simulink subsystem "Simulation"  (R2025b)
settings: Solver=VariableStepAuto  StartTime=0.0  StopTime=10.0  RelTol=1e-3
undefined symbols (not defined in the file or in its folder): angular_velocity, AUV, data, data_SL_Info, elevation, fractalcoef, heading, height, linear_acceleration, orientation, Sim3dSensor, Simple, T200, thruster_pose, width, x_vel_btm, XYZ, y_vel_btm, z_vel_btm
libraries: ros2lib x15, sim3dlib x7, robotcorelib x5, AUVLib x4, aerolib6dof2 x2, sim3dcameralib x2, matrix_library x1, mspsensorlib x1, aerolibutil x1, mspfiltlib x1
(part 1 of 2)
settings Model: Creator=ubuntu  LastModifiedBy=ubuntu

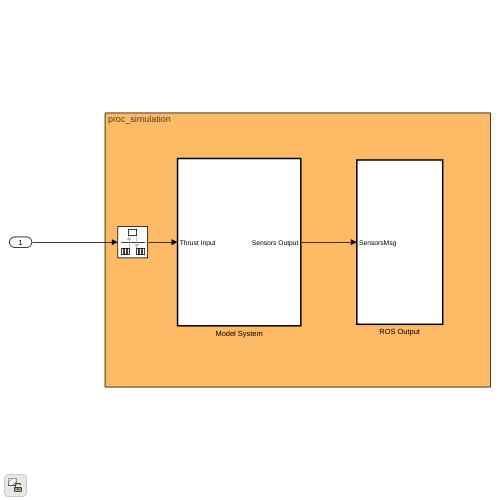
[thumbnail: Simulink's stored preview of the top-level diagram]
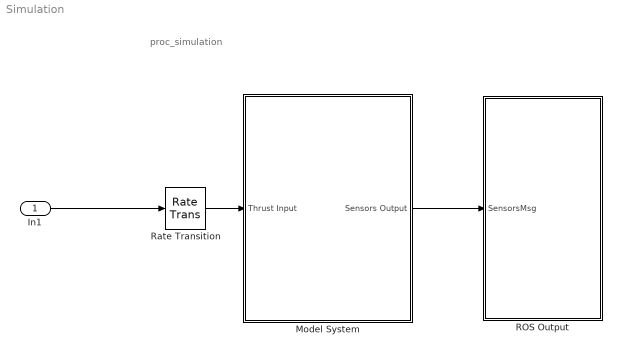
== system Simulation ==
  note: proc_simulation
  In1 : Inport
  Model System : Subsystem  TreatAsAtomicUnit=on
  ROS Output : Subsystem  TreatAsAtomicUnit=on
  Rate Transition : RateTransition  OutPortSampleTime=0.05
  wires:
  Model System/1(Sensors Output) -> ROS Output/1(SensorsMsg)
  In1/1 -> Rate Transition/1
  Rate Transition/1 -> Model System/1(Thrust Input)

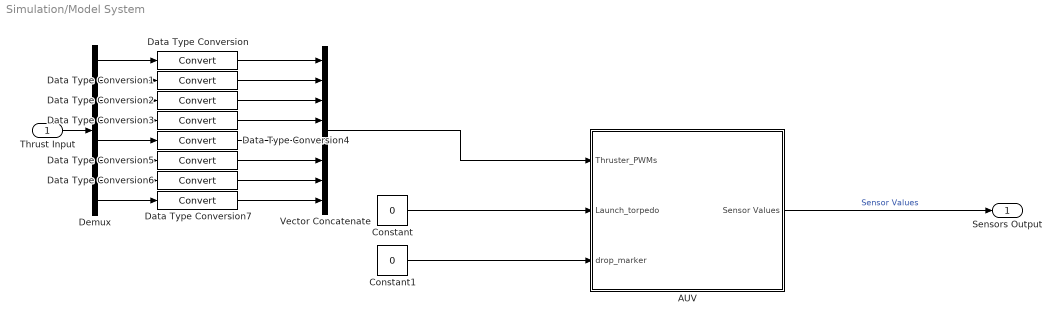
== system Simulation/Model System ==
  Thrust Input : Inport
  AUV : Subsystem  mask(RoboSub){SourceFile=./src/virtual-robosub/fbx files/AUV2.stl, AUV_cob=[0.01, -0.02, -0.10], AUV_height=AUV.Body.hulldiameter, AUV_vol=0.0365, AUV_inertia=AUV.Body.Inertia, AUV_mass=31.42, AUV_pos=[-142 -142 -1], AUV_orientation=[0 0 pi/2], thruster_pose=thruster_pose, AUV_Voltage=16V, nThrusters=8, Hy=Simple, lin_coeff=diag([ 150,200,153]), quad_coeff=diag([ 11.7, 8.2, 7.56]), ang_coeff=diag([ 33, 23, 50]), CMK=AUV.Coeff.CMM, CMM=AUV.Coeff.CMN, CMN=AUV.Coeff.CMK, CZ=AUV.Coeff.CZ, CY=AUV.Coeff.CY, CX=AUV.Coeff.CX, betaR=AUV.IncRange.beta_vec, alphaR=AUV.IncRange.alpha_vec, ang_coeff_c=diag([10, 80, 80]), d_cam_pos=[0 0 -0.26], d_orientation=[0 90 0], SemanticOutportEnabled=off, DepthOutportEnabled=off, TangentialDistortion=[0, 0], RadialDistortion=[0, 0], ImageSize=[720, 1280], OpticalCenter=[640, 360], FocalLength=[1109, 1109], f_cam_pos=[0.5, 0, 0], f_orientation=[0 0 0], SemanticOutportEnabled_f=off, DepthOutportEnabled_f=on, TangentialDistortion_f=[0, 0], RadialDistortion_f=[0, 0], ImageSize_f=[720, 1280], OpticalCenter_f=[640, 360], FocalLength_f=[1109, 1109], ref_mode=Bottom Tracking, Temperature=25, MagneticFieldNED=XYZ, AccelParamsMeasurementRange=Inf, AccelParamsResolution=0, AccelParamsConstantBias=[ 0, 0, 0 ], AccelParamsAxesMisalignment=[ 100, 0, 0; 0, 100, 0; 0, 0, 100 ], AccelParamsNoiseDensity=[ 0, 0, 0 ], AccelParamsBiasInstability=[ 0, 0, 0 ], AccelParamsBiasInstabilityNumerator=fractalcoef().Numerator, AccelParamsBiasInstabilityDenominator=fractalcoef().Denominator, AccelParamsRandomWalk=[ 0, 0, 0 ], AccelParamsNoiseType=double-sided, AccelParamsTemperatureBias=[ 0, 0, 0 ], AccelParamsTemperatureScaleFactor=[ 0, 0, 0 ], GyroParamsMeasurementRange=Inf, GyroParamsResolution=0, GyroParamsConstantBias=[ 0, 0, 0 ], GyroParamsAxesMisalignment=[ 100, 0, 0; 0, 100, 0; 0, 0, 100 ], GyroParamsAccelerationBias=[ 0, 0, 0 ], GyroParamsNoiseDensity=[ 0, 0, 0 ], GyroParamsBiasInstability=[ 0, 0, 0 ], GyroParamsBiasInstabilityNumerator=fractalcoef().Numerator, GyroParamsBiasInstabilityDenominator=fractalcoef().Denominator, GyroParamsRandomWalk=[ 0, 0, 0 ], GyroParamsNoiseType=double-sided, GyroParamsTemperatureBias=[ 0, 0, 0 ], GyroParamsTemperatureScaleFactor=[ 0, 0, 0 ], MagParamsMeasurementRange=Inf, MagParamsResolution=0, MagParamsConstantBias=[ 0, 0, 0 ], MagParamsAxesMisalignment=[ 100, 0, 0; 0, 100, 0; 0, 0, 100 ], MagParamsNoiseDensity=[ 0, 0, 0 ], MagParamsBiasInstability=[ 0, 0, 0 ], MagParamsBiasInstabilityNumerator=fractalcoef().Numerator, MagParamsBiasInstabilityDenominator=fractalcoef().Denominator, MagParamsRandomWalk=[ 0, 0, 0 ], MagParamsNoiseType=double-sided, MagParamsTemperatureBias=[ 0, 0, 0 ], MagParamsTemperatureScaleFactor=[ 0, 0, 0 ], torp_pos=[0.4 0.2 0.1], marker_pos=[-0.01 0 0.02], waterDensity=1000, gravity=9.79624, w_current=None, waterCurrent=[0 0 0], causticsVisibility=off}
      mask prompts: SourceFile "Path to AUV model"; AUV_cob "CoB (relative to CoM) (m)"; AUV_height "Height (or diameter) of AUV (m)"; AUV_vol "Volume of AUV (m^3)"; AUV_inertia "Inerita matrix of AUV"; AUV_mass "Mass of AUV (kg)"; AUV_pos "Inital Position [x,y,z] (m)"; AUV_orientation "Inital Euler Orientation [roll, pith, yaw] (rad)"; thruster_pose "Thruster Pose (nx6 matrix) (m,rad)"; AUV_Voltage "AUV Battery Voltage"; nThrusters "Number of thrusters"; Hy "Choose Hydrodynamics Simulation"; lin_coeff "Linear drag coefficient"; quad_coeff "Quadratic drag coefficient"; ang_coeff "Angular Damping coefficient"; CMK "Rolling moment coeff"; CMM "Pitching moment coeff"; CMN "Yawing moment coeff"; CZ "Normal force coeff (CZ)"; CY "Side force coeff (CY)"; CX "Axial force coeff (CX)"; betaR "Beta Range"; alphaR "Alpha Range"; ang_coeff_c "Angular Damping coefficient"; d_cam_pos "Position (relative to CoM) (m)"; d_orientation "Orientation (deg)"; SemanticOutportEnabled "shared_sim3dblks:sim3dblkCameraPinHole:blkPrm_SemanticOutportEnabled"; DepthOutportEnabled "shared_sim3dblks:sim3dblkCameraPinHole:blkPrm_DepthOutportEnabled"; TangentialDistortion "shared_sim3dblks:sim3dblkCameraPinHole:blkPrm_TangentialDistortion"; RadialDistortion "shared_sim3dblks:sim3dblkCameraPinHole:blkPrm_RadialDistortion"; ImageSize "shared_sim3dblks:sim3dblkCameraPinHole:blkPrm_ImageSize"; OpticalCenter "shared_sim3dblks:sim3dblkCameraPinHole:blkPrm_OpticalCenter"; FocalLength "shared_sim3dblks:sim3dblkCameraPinHole:blkPrm_FocalLength"; f_cam_pos "Position (relative to CoM) (m)"; f_orientation "Orientation (deg)"; SemanticOutportEnabled_f "shared_sim3dblks:sim3dblkCameraPinHole:blkPrm_SemanticOutportEnabled"; DepthOutportEnabled_f "shared_sim3dblks:sim3dblkCameraPinHole:blkPrm_DepthOutportEnabled"; TangentialDistortion_f "shared_sim3dblks:sim3dblkCameraPinHole:blkPrm_TangentialDistortion"; RadialDistortion_f "shared_sim3dblks:sim3dblkCameraPinHole:blkPrm_RadialDistortion"; ImageSize_f "shared_sim3dblks:sim3dblkCameraPinHole:blkPrm_ImageSize"; OpticalCenter_f "shared_sim3dblks:sim3dblkCameraPinHole:blkPrm_OpticalCenter"; FocalLength_f "shared_sim3dblks:sim3dblkCameraPinHole:blkPrm_FocalLength"; ref_mode "Reference mode"; Temperature "Temperature (°C):"; MagneticFieldNED "Magnetic field (NED):"; AccelParamsMeasurementRange "Maximum readings (m/s²):"; AccelParamsResolution "Resolution ((m/s²)/LSB):"; AccelParamsConstantBias "Constant offset bias (m/s²):"; AccelParamsAxesMisalignment "Axes skew (%):"; AccelParamsNoiseDensity "Velocity random walk ((m/s²)/√Hz):"; AccelParamsBiasInstability "Bias instability (m/s²):"; AccelParamsBiasInstabilityNumerator "Bias instability filter numerator coefficients:"; AccelParamsBiasInstabilityDenominator "Bias instability filter denominator coefficients:"; AccelParamsRandomWalk "Acceleration random walk ((m/s²)*√Hz):"; AccelParamsNoiseType "Noise type:"; AccelParamsTemperatureBias "Bias from temperature ((m/s²)/°C):"; AccelParamsTemperatureScaleFactor "Temperature scale factor (%/°C):"; GyroParamsMeasurementRange "Maximum readings (rad/s):"; GyroParamsResolution "Resolution ((rad/s)/LSB):"; GyroParamsConstantBias "Constant offset bias (rad/s):"; GyroParamsAxesMisalignment "Axes skew (%):"; GyroParamsAccelerationBias "Bias from acceleration ((rad/s)/(m/s²)):"; GyroParamsNoiseDensity "Angle random walk ((rad/s)/√Hz):"; GyroParamsBiasInstability "Bias instability (rad/s):"; GyroParamsBiasInstabilityNumerator "Bias instability filter numerator coefficients:"; GyroParamsBiasInstabilityDenominator "Bias instability filter denominator coefficients:"; GyroParamsRandomWalk "Rate random walk ((rad/s)*√Hz):"; GyroParamsNoiseType "Noise type:"; GyroParamsTemperatureBias "Bias from temperature ((rad/s)/°C):"; GyroParamsTemperatureScaleFactor "Temperature scale factor (%/°C):"; MagParamsMeasurementRange "Maximum readings (µT):"; MagParamsResolution "Resolution ((µT)/LSB):"; MagParamsConstantBias "Constant offset bias (µT):"; MagParamsAxesMisalignment "Axes skew (%):"; MagParamsNoiseDensity "White Noise PSD ((µT)/√Hz):"; MagParamsBiasInstability "Bias instability (µT):"; MagParamsBiasInstabilityNumerator "Bias instability filter numerator coefficients:"; MagParamsBiasInstabilityDenominator "Bias instability filter denominator coefficients:"; MagParamsRandomWalk "Random walk ((µT)*√Hz):"; MagParamsNoiseType "Noise type:"; MagParamsTemperatureBias "Bias from temperature ((µT)/°C):"; MagParamsTemperatureScaleFactor "Temperature scale factor (%/°C):"; torp_pos "Torpedo position (m)"; marker_pos "marker_pos (m)"; waterDensity "Water Density (kg/m^3)"; gravity "Acceleration due to Gravity (m/sec^2)"; w_current "Water current"; waterCurrent "Enter current speed in x and y (z=0) (m/s)"; causticsVisibility "Enable Water Caustics"
      mask help:
      | The mask takes in necessary information required to simulate the AUV in a pool. It is divided into 4 sections - AUV Parameters, Sensors, Actuators and Environment.
      | The AUV Parameters section contains all the data related to the AUV body such as mass, inertia, volume, etc. It also takes in the hydrodynamic coefficients (based on the chosen complexity).
      | The Sensors section takes in data related to the sensors such as mounting location and any sensor parameters (for ex: camera - focal lenght, resolution, distortions, etc.)
      | The Actuators sections takes in the mounting location for 2 actuators present in the simulator - torpedo and marker.
      | The Environment section has some parameters related of the environment such as water density, gravity and water currents.
      mask TypeOptions SourceFile: Visualization/AUV mesh/SourceFile
      mask TypeOptions Hy: AUV Dynamics/Environmental Forces and Moments/Hy
      mask TypeOptions lin_coeff: AUV Dynamics/Environmental Forces and Moments/lin_coeff
      mask TypeOptions quad_coeff: AUV Dynamics/Environmental Forces and Moments/quad_coeff
      mask TypeOptions ang_coeff: AUV Dynamics/Environmental Forces and Moments/ang_coeff
      mask TypeOptions CMK: AUV Dynamics/Environmental Forces and Moments/CMK
      mask TypeOptions CMM: AUV Dynamics/Environmental Forces and Moments/CMM
      mask TypeOptions CMN: AUV Dynamics/Environmental Forces and Moments/CMN
      mask TypeOptions CZ: AUV Dynamics/Environmental Forces and Moments/CZ
      mask TypeOptions CY: AUV Dynamics/Environmental Forces and Moments/CY
      mask TypeOptions CX: AUV Dynamics/Environmental Forces and Moments/CX
      mask TypeOptions betaR: AUV Dynamics/Environmental Forces and Moments/betaR
      mask TypeOptions alphaR: AUV Dynamics/Environmental Forces and Moments/alphaR
      mask TypeOptions ang_coeff_c: AUV Dynamics/Environmental Forces and Moments/ang_coeff_c
      mask TypeOptions SemanticOutportEnabled: Sensors/downward_camera/SemanticOutportEnabled
      mask TypeOptions DepthOutportEnabled: Sensors/downward_camera/DepthOutportEnabled
      mask TypeOptions TangentialDistortion: Sensors/downward_camera/TangentialDistortion
      mask TypeOptions RadialDistortion: Sensors/downward_camera/RadialDistortion
      mask TypeOptions ImageSize: Sensors/downward_camera/ImageSize
      mask TypeOptions OpticalCenter: Sensors/downward_camera/OpticalCenter
      mask TypeOptions FocalLength: Sensors/downward_camera/FocalLength
      mask TypeOptions SemanticOutportEnabled_f: Sensors/forward_camera/SemanticOutportEnabled
      mask TypeOptions DepthOutportEnabled_f: Sensors/forward_camera/DepthOutportEnabled
      mask TypeOptions TangentialDistortion_f: Sensors/forward_camera/TangentialDistortion
      mask TypeOptions RadialDistortion_f: Sensors/forward_camera/RadialDistortion
      mask TypeOptions ImageSize_f: Sensors/forward_camera/ImageSize
      mask TypeOptions OpticalCenter_f: Sensors/forward_camera/OpticalCenter
      mask TypeOptions FocalLength_f: Sensors/forward_camera/FocalLength
      mask TypeOptions Temperature: Sensors/IMU Subsystem/IMU/Temperature
      mask TypeOptions MagneticFieldNED: Sensors/IMU Subsystem/IMU/MagneticFieldNED
      mask TypeOptions AccelParamsMeasurementRange: Sensors/IMU Subsystem/IMU/AccelParamsMeasurementRange
      mask TypeOptions AccelParamsResolution: Sensors/IMU Subsystem/IMU/AccelParamsResolution
      mask TypeOptions AccelParamsConstantBias: Sensors/IMU Subsystem/IMU/AccelParamsConstantBias
      mask TypeOptions AccelParamsAxesMisalignment: Sensors/IMU Subsystem/IMU/AccelParamsAxesMisalignment
      mask TypeOptions AccelParamsNoiseDensity: Sensors/IMU Subsystem/IMU/AccelParamsNoiseDensity
      mask TypeOptions AccelParamsBiasInstability: Sensors/IMU Subsystem/IMU/AccelParamsBiasInstability
      mask TypeOptions AccelParamsBiasInstabilityNumerator: Sensors/IMU Subsystem/IMU/AccelParamsBiasInstabilityNumerator
      mask TypeOptions AccelParamsBiasInstabilityDenominator: Sensors/IMU Subsystem/IMU/AccelParamsBiasInstabilityDenominator
      mask TypeOptions AccelParamsRandomWalk: Sensors/IMU Subsystem/IMU/AccelParamsRandomWalk
      mask TypeOptions AccelParamsNoiseType: Sensors/IMU Subsystem/IMU/AccelParamsNoiseType
      mask TypeOptions AccelParamsTemperatureBias: Sensors/IMU Subsystem/IMU/AccelParamsTemperatureBias
      mask TypeOptions AccelParamsTemperatureScaleFactor: Sensors/IMU Subsystem/IMU/AccelParamsTemperatureScaleFactor
      mask TypeOptions GyroParamsMeasurementRange: Sensors/IMU Subsystem/IMU/GyroParamsMeasurementRange
      mask TypeOptions GyroParamsResolution: Sensors/IMU Subsystem/IMU/GyroParamsResolution
      mask TypeOptions GyroParamsConstantBias: Sensors/IMU Subsystem/IMU/GyroParamsConstantBias
      mask TypeOptions GyroParamsAxesMisalignment: Sensors/IMU Subsystem/IMU/GyroParamsAxesMisalignment
      mask TypeOptions GyroParamsAccelerationBias: Sensors/IMU Subsystem/IMU/GyroParamsAccelerationBias
      mask TypeOptions GyroParamsNoiseDensity: Sensors/IMU Subsystem/IMU/GyroParamsNoiseDensity
      mask TypeOptions GyroParamsBiasInstability: Sensors/IMU Subsystem/IMU/GyroParamsBiasInstability
      mask TypeOptions GyroParamsBiasInstabilityNumerator: Sensors/IMU Subsystem/IMU/GyroParamsBiasInstabilityNumerator
      mask TypeOptions GyroParamsBiasInstabilityDenominator: Sensors/IMU Subsystem/IMU/GyroParamsBiasInstabilityDenominator
      mask TypeOptions GyroParamsRandomWalk: Sensors/IMU Subsystem/IMU/GyroParamsRandomWalk
      mask TypeOptions GyroParamsNoiseType: Sensors/IMU Subsystem/IMU/GyroParamsNoiseType
      mask TypeOptions GyroParamsTemperatureBias: Sensors/IMU Subsystem/IMU/GyroParamsTemperatureBias
      mask TypeOptions GyroParamsTemperatureScaleFactor: Sensors/IMU Subsystem/IMU/GyroParamsTemperatureScaleFactor
      mask TypeOptions MagParamsMeasurementRange: Sensors/IMU Subsystem/IMU/MagParamsMeasurementRange
      mask TypeOptions MagParamsResolution: Sensors/IMU Subsystem/IMU/MagParamsResolution
      mask TypeOptions MagParamsConstantBias: Sensors/IMU Subsystem/IMU/MagParamsConstantBias
      mask TypeOptions MagParamsAxesMisalignment: Sensors/IMU Subsystem/IMU/MagParamsAxesMisalignment
      mask TypeOptions MagParamsNoiseDensity: Sensors/IMU Subsystem/IMU/MagParamsNoiseDensity
      mask TypeOptions MagParamsBiasInstability: Sensors/IMU Subsystem/IMU/MagParamsBiasInstability
      mask TypeOptions MagParamsBiasInstabilityNumerator: Sensors/IMU Subsystem/IMU/MagParamsBiasInstabilityNumerator
      mask TypeOptions MagParamsBiasInstabilityDenominator: Sensors/IMU Subsystem/IMU/MagParamsBiasInstabilityDenominator
      mask TypeOptions MagParamsRandomWalk: Sensors/IMU Subsystem/IMU/MagParamsRandomWalk
      mask TypeOptions MagParamsNoiseType: Sensors/IMU Subsystem/IMU/MagParamsNoiseType
      mask TypeOptions MagParamsTemperatureBias: Sensors/IMU Subsystem/IMU/MagParamsTemperatureBias
      mask TypeOptions MagParamsTemperatureScaleFactor: Sensors/IMU Subsystem/IMU/MagParamsTemperatureScaleFactor
      mask DialogControl Container3 Prompt: AUV Parameters
      mask DialogControl Container4 Prompt: General
      mask DialogControl Container5 Prompt: Hydrodynamics
      mask DialogControl Container6 Prompt: Simple hydrodynamics coefficients
      mask DialogControl Container7 Prompt: Complex hydrodynamics coefficients
      mask DialogControl Container8 Prompt: Sensors
      mask DialogControl Container10 Prompt: Downward Camera
      mask DialogControl SemanticOutportEnabled Prompt: Output semantic segmentation
      mask DialogControl DepthOutportEnabled Prompt: Output depth
      mask DialogControl TangentialDistortion Prompt: Tangential distortion coefficients:
      mask DialogControl RadialDistortion Prompt: Radial distortion coefficients:
      mask DialogControl ImageSize Prompt: Image size (pixels):
      mask DialogControl OpticalCenter Prompt: Optical center (pixels):
      mask DialogControl FocalLength Prompt: Focal length (pixels):
      mask DialogControl Container9 Prompt: Forward Camera
      mask DialogControl SemanticOutportEnabled_f Prompt: Output semantic segmentation
      mask DialogControl DepthOutportEnabled_f Prompt: Output depth
      mask DialogControl TangentialDistortion_f Prompt: Tangential distortion coefficients:
      mask DialogControl RadialDistortion_f Prompt: Radial distortion coefficients:
      mask DialogControl ImageSize_f Prompt: Image size (pixels):
      mask DialogControl OpticalCenter_f Prompt: Optical center (pixels):
      mask DialogControl FocalLength_f Prompt: Focal length (pixels):
      mask DialogControl Container11 Prompt: DVL
      mask DialogControl Container12 Prompt: IMU
      mask DialogControl Container16 Prompt: Accelerometer
      mask DialogControl Container17 Prompt: Gyroscope
      mask DialogControl Container18 Prompt: Magnetometer
      mask DialogControl Container13 Prompt: Actuators
      mask DialogControl Container14 Prompt: Environment
      mask Display: image('submarine.png');
  Constant : Constant  Value=0
  Constant1 : Constant  Value=0
  Data Type Conversion{,1..7} (8 alike) : DataTypeConversion  SaturateOnIntegerOverflow=off  RndMeth=Floor
  Demux : Demux  Outputs=8
  Vector Concatenate : Concatenate  NumInputs=8
  Sensors Output : Outport
  wires:
  Demux/8 -> Data Type Conversion7/1
  Demux/7 -> Data Type Conversion6/1
  Demux/6 -> Data Type Conversion5/1
  Demux/5 -> Data Type Conversion4/1
  Demux/4 -> Data Type Conversion3/1
  Demux/3 -> Data Type Conversion2/1
  Demux/2 -> Data Type Conversion1/1
  Demux/1 -> Data Type Conversion/1
  Data Type Conversion3/1 -> Vector Concatenate/4
  Data Type Conversion2/1 -> Vector Concatenate/3
  Data Type Conversion1/1 -> Vector Concatenate/2
  Data Type Conversion/1 -> Vector Concatenate/1
  Data Type Conversion7/1 -> Vector Concatenate/8
  Data Type Conversion6/1 -> Vector Concatenate/7
  Data Type Conversion5/1 -> Vector Concatenate/6
  Data Type Conversion4/1 -> Vector Concatenate/5
  Vector Concatenate/1 -> AUV/1(Thruster_PWMs)
  AUV/1(Sensor Values) -> Sensors Output/1  "Sensor Values"
  Constant/1 -> AUV/2(Launch_torpedo)
  Constant1/1 -> AUV/3(drop_marker)
  Thrust Input/1 -> Demux/1

== system Simulation/ROS Output ==
  note: Sensor msg
  SensorsMsg : Inport
  Send DVL msg : Subsystem
  Send Depth msg : Subsystem
  Send Depth msg1 : Subsystem
  Send IMU Msg : Subsystem
  Send Ping msg : Subsystem  Commented=on
  wires:
  SensorsMsg/1 -> Send IMU Msg/1(Response), Send DVL msg/1(Response), Send Depth msg/1(Mesure), Send Ping msg/1(Mesure), Send Depth msg1/1(Mesure)

== system Simulation/Model System/AUV ==
  Thruster_PWMs : Inport
  Launch_torpedo : Inport  Port=2
  drop_marker : Inport  Port=3
  AUV Dynamics : Subsystem
  Actuators : Subsystem
  Sensors : Subsystem
  Visualization : Subsystem
  Sensor Values : Outport
  wires:
  Actuators/2(marker_position) -> Visualization/3(Marker Position)
  Actuators/1(Torpedo Pose) -> Visualization/2(Torpedo Pose)
  drop_marker/1 -> Actuators/3(drop_marker)
  Launch_torpedo/1 -> Actuators/2(Launch_torpedo)
  AUV Dynamics/1(Robot State) -> Visualization/1(Robot State), Actuators/1(Robot State), Sensors/1(Robot State)
  Sensors/1(Sensor Values) -> Sensor Values/1
  Thruster_PWMs/1 -> AUV Dynamics/1(Thruster_PWMs)

== system Simulation/ROS Output/Send DVL msg ==
  Response : Inport
  Blank Message : ros2lib/Blank Message  messageClass=Message  entityType=sonia_common_ros2/BodyVelocityDVL  messageType=sonia_common_ros2/BodyVelocityDVL  SampleTime=inf
  Bus Assignment : BusAssignment  AssignedSignals=x_vel_btm,y_vel_btm,z_vel_btm
  Bus Selector : BusSelector  OutputSignals=vel_b_dvl
  Demux : Demux  Outputs=3
  Gain : Gain  Gain=-1
  Publish : ros2lib/Publish  topicSource=Specify your own  topic=/proc_simulation/dvl_velocity  messageType=sonia_common_ros2/BodyVelocityDVL  QOSHistory=Keep last  QOSDepth=1  QOSReliability=Reliable  QOSDurability=Volatile  QOSDeadline=Inf  QOSLifespan=Inf  QOSLiveliness=Automatic  QOSLeaseDuration=Inf  QOSAvoidROSNamespaceConventions=off
  Rate Transition : RateTransition  OutPortSampleTime=0.1
  wires:
  Rate Transition/1 -> Bus Selector/1
  Gain/1 -> Bus Assignment/4
  Demux/1 -> Bus Assignment/2
  Demux/2 -> Bus Assignment/3
  Demux/3 -> Gain/1
  Bus Assignment/1 -> Publish/1
  Blank Message/1 -> Bus Assignment/1
  Bus Selector/1 -> Demux/1  "<vel_b_dvl>"
  Response/1 -> Rate Transition/1

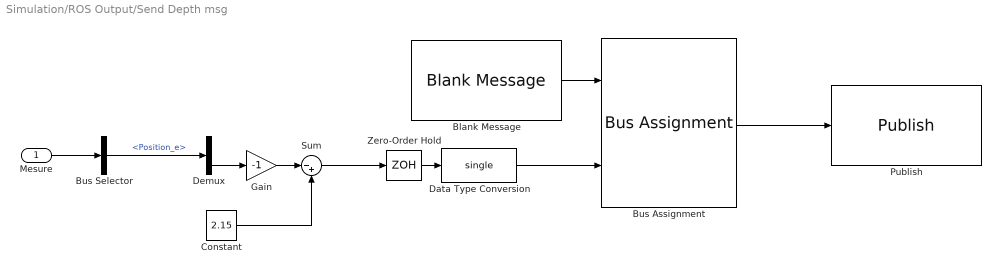
== system Simulation/ROS Output/Send Depth msg ==
  Mesure : Inport
  Blank Message : ros2lib/Blank Message  messageClass=Message  entityType=std_msgs/Float32  messageType=std_msgs/Float32  SampleTime=inf
  Bus Assignment : BusAssignment  AssignedSignals=data
  Bus Selector : BusSelector  OutputSignals=Position_e
  Constant : Constant  Value=2.15
  Data Type Conversion : DataTypeConversion  OutDataTypeStr=single  SaturateOnIntegerOverflow=off  RndMeth=Floor
  Demux : Demux  Outputs=3
  Gain : Gain  Gain=-1
  Publish : ros2lib/Publish  topicSource=Specify your own  topic=/proc_simulation/depth  messageType=std_msgs/Float32  QOSHistory=Keep last  QOSDepth=1  QOSReliability=Reliable  QOSDurability=Volatile  QOSDeadline=Inf  QOSLifespan=Inf  QOSLiveliness=Automatic  QOSLeaseDuration=Inf  QOSAvoidROSNamespaceConventions=off
  Sum : Sum  Inputs=|-+
  Zero-Order Hold : ZeroOrderHold  SampleTime=simulation.sensors.depth.sampletime
  wires:
  Mesure/1 -> Bus Selector/1
  Gain/1 -> Sum/1
  Constant/1 -> Sum/2
  Sum/1 -> Zero-Order Hold/1
  Demux/3 -> Gain/1
  Bus Assignment/1 -> Publish/1
  Blank Message/1 -> Bus Assignment/1
  Bus Selector/1 -> Demux/1  "<Position_e>"
  Zero-Order Hold/1 -> Data Type Conversion/1
  Data Type Conversion/1 -> Bus Assignment/2

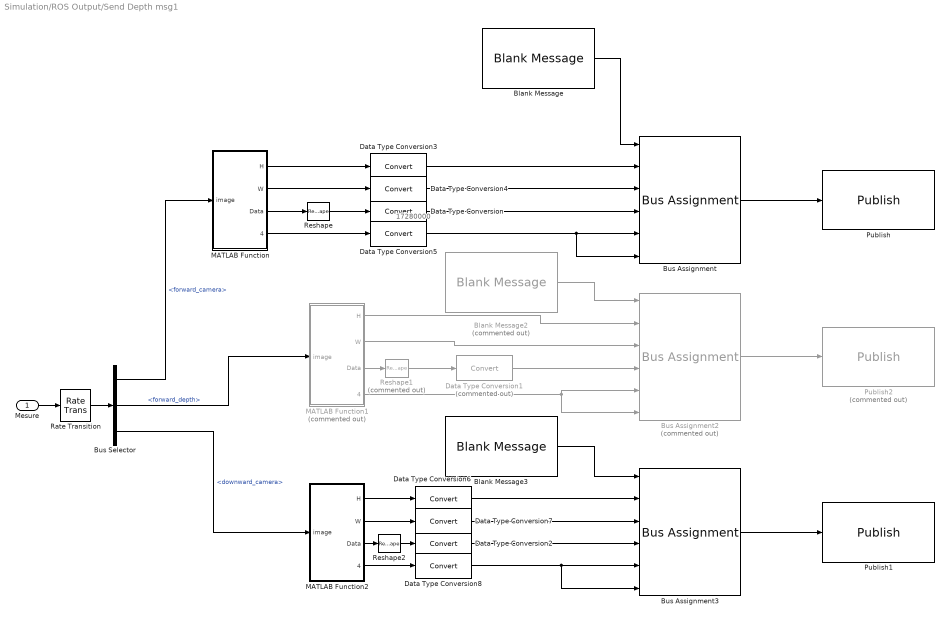
== system Simulation/ROS Output/Send Depth msg1 ==
  note: 17280000
  Mesure : Inport
  Blank Message : ros2lib/Blank Message  messageClass=Message  entityType=sensor_msgs/Image  messageType=sensor_msgs/Image  SampleTime=inf
  Blank Message2 : ros2lib/Blank Message  Commented=on  messageClass=Message  entityType=sensor_msgs/Image  messageType=sensor_msgs/Image  SampleTime=inf
  Blank Message3 : ros2lib/Blank Message  messageClass=Message  entityType=sensor_msgs/Image  messageType=sensor_msgs/Image  SampleTime=inf
  Bus Assignment : BusAssignment  AssignedSignals=height,width,data,data_SL_Info.CurrentLength,data_SL_Info.ReceivedLength
  Bus Assignment2 : BusAssignment  Commented=on  AssignedSignals=height,width,data,data_SL_Info.CurrentLength,data_SL_Info.ReceivedLength
  Bus Assignment3 : BusAssignment  AssignedSignals=height,width,data,data_SL_Info.CurrentLength,data_SL_Info.ReceivedLength
  Bus Selector : BusSelector  OutputSignals=forward_camera,forward_depth,downward_camera
  Data Type Conversion{,2..8} (8 alike) : DataTypeConversion  SaturateOnIntegerOverflow=off  RndMeth=Floor
  Data Type Conversion1 : DataTypeConversion  Commented=on  SaturateOnIntegerOverflow=off  RndMeth=Floor
  MATLAB Function : MATLAB Function  TreatAsAtomicUnit=on
  MATLAB Function1 : MATLAB Function  Commented=on  TreatAsAtomicUnit=on
  MATLAB Function2 : MATLAB Function  TreatAsAtomicUnit=on
  Publish : ros2lib/Publish  topicSource=Specify your own  topic=/proc_simulation/front  messageType=sensor_msgs/Image  QOSHistory=Keep last  QOSDepth=1  QOSReliability=Reliable  QOSDurability=Volatile  QOSDeadline=Inf  QOSLifespan=Inf  QOSLiveliness=Automatic  QOSLeaseDuration=Inf  QOSAvoidROSNamespaceConventions=off
  Publish1 : ros2lib/Publish  topicSource=Specify your own  topic=/proc_simulation/bottom  messageType=sensor_msgs/Image  QOSHistory=Keep last  QOSDepth=1  QOSReliability=Reliable  QOSDurability=Volatile  QOSDeadline=Inf  QOSLifespan=Inf  QOSLiveliness=Automatic  QOSLeaseDuration=Inf  QOSAvoidROSNamespaceConventions=off
  Publish2 : ros2lib/Publish  Commented=on  topicSource=Specify your own  topic=/proc_simulation/front  messageType=sensor_msgs/Image  QOSHistory=Keep last  QOSDepth=1  QOSReliability=Reliable  QOSDurability=Volatile  QOSDeadline=Inf  QOSLifespan=Inf  QOSLiveliness=Automatic  QOSLeaseDuration=Inf  QOSAvoidROSNamespaceConventions=off
  Rate Transition : RateTransition  OutPortSampleTime=0.1
  Reshape : Reshape
  Reshape1 : Reshape  Commented=on
  Reshape2 : Reshape
  wires:
  Rate Transition/1 -> Bus Selector/1
  Data Type Conversion8/1 -> Bus Assignment3/5, Bus Assignment3/6
  Data Type Conversion7/1 -> Bus Assignment3/3
  Data Type Conversion6/1 -> Bus Assignment3/2
  Data Type Conversion5/1 -> Bus Assignment/5, Bus Assignment/6
  Data Type Conversion4/1 -> Bus Assignment/3
  Data Type Conversion3/1 -> Bus Assignment/2
  Reshape2/1 -> Data Type Conversion2/1
  Reshape1/1 -> Data Type Conversion1/1
  Reshape/1 -> Data Type Conversion/1
  Data Type Conversion2/1 -> Bus Assignment3/4
  Data Type Conversion1/1 -> Bus Assignment2/4
  Data Type Conversion/1 -> Bus Assignment/4
  Bus Selector/3 -> MATLAB Function2/1(image)  "<downward_camera>"
  Bus Assignment3/1 -> Publish1/1
  MATLAB Function2/2(W) -> Data Type Conversion7/1
  MATLAB Function2/1(H) -> Data Type Conversion6/1
  MATLAB Function2/4(DataLength) -> Data Type Conversion8/1
  Blank Message3/1 -> Bus Assignment3/1
  MATLAB Function2/3(Data) -> Reshape2/1
  MATLAB Function1/3(Data) -> Reshape1/1
  MATLAB Function1/2(W) -> Bus Assignment2/3
  MATLAB Function1/1(H) -> Bus Assignment2/2
  MATLAB Function1/4(DataLength) -> Bus Assignment2/6, Bus Assignment2/5
  MATLAB Function/4(DataLength) -> Data Type Conversion5/1
  MATLAB Function/3(Data) -> Reshape/1
  MATLAB Function/2(W) -> Data Type Conversion4/1
  MATLAB Function/1(H) -> Data Type Conversion3/1
  Bus Assignment2/1 -> Publish2/1
  Bus Selector/2 -> MATLAB Function1/1(image)  "<forward_depth>"
  Blank Message2/1 -> Bus Assignment2/1
  Bus Selector/1 -> MATLAB Function/1(image)  "<forward_camera>"
  Bus Assignment/1 -> Publish/1
  Blank Message/1 -> Bus Assignment/1
  Mesure/1 -> Rate Transition/1

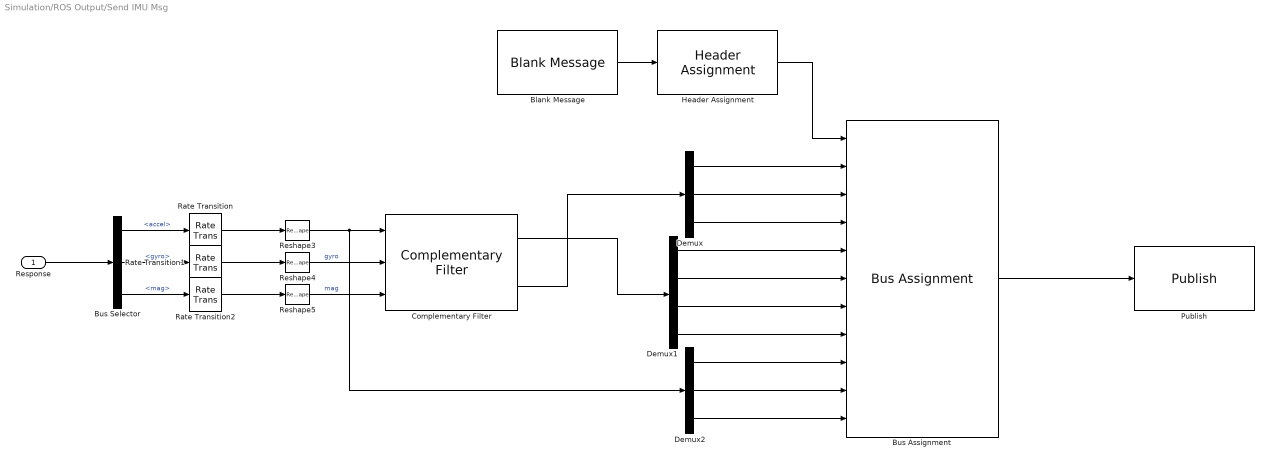
== system Simulation/ROS Output/Send IMU Msg ==
  Response : Inport
  Blank Message : ros2lib/Blank Message  messageClass=Message  entityType=sensor_msgs/Imu  messageType=sensor_msgs/Imu  SampleTime=inf
  Bus Assignment : BusAssignment  AssignedSignals=angular_velocity.x,angular_velocity.y,angular_velocity.z,orientation.w,orientation.x,orientation.y,orientation.z,linear_acceleration.x,linear_acceleration.y,linear_acceleration.z
  Bus Selector : BusSelector  OutputSignals=accel,gyro,mag
  Complementary Filter : mspfiltlib/Complementary Filter  DispRefFrame=NED  OrientationFormat=quaternion  AccelerometerGain=0.02  HasMagnetometer=on  MagnetometerGain=0.02  SimulateUsing=Interpreted execution
  Demux : Demux  Outputs=3
  Demux1 : Demux
  Demux2 : Demux  Outputs=3
  Header Assignment : ros2lib/Header Assignment  SetFrameID=on  FrameID=NED  InsertTimeStamp=on  SetHeaderFieldName=Use the default header field name  HeaderFieldName=header
  Publish : ros2lib/Publish  topicSource=Specify your own  topic=/proc_simulation/imu_info  messageType=sensor_msgs/Imu  QOSHistory=Keep last  QOSDepth=1  QOSReliability=Reliable  QOSDurability=Volatile  QOSDeadline=Inf  QOSLifespan=Inf  QOSLiveliness=Automatic  QOSLeaseDuration=Inf  QOSAvoidROSNamespaceConventions=off
  Rate Transition : RateTransition  OutPortSampleTime=0.02
  Rate Transition1 : RateTransition  OutPortSampleTime=0.02
  Rate Transition2 : RateTransition  OutPortSampleTime=0.02
  Reshape3 : Reshape  OutputDimensionality=Row vector (2-D)
  Reshape4 : Reshape  OutputDimensionality=Row vector (2-D)
  Reshape5 : Reshape  OutputDimensionality=Row vector (2-D)
  wires:
  Demux/2 -> Bus Assignment/3
  Demux1/3 -> Bus Assignment/7
  Rate Transition2/1 -> Reshape5/1
  Rate Transition1/1 -> Reshape4/1
  Rate Transition/1 -> Reshape3/1
  Response/1 -> Bus Selector/1
  Reshape5/1 -> Complementary Filter/3  "mag"
  Reshape4/1 -> Complementary Filter/2  "gyro"
  Reshape3/1 -> Demux2/1, Complementary Filter/1
  Complementary Filter/2 -> Demux/1
  Complementary Filter/1 -> Demux1/1
  Bus Selector/3 -> Rate Transition2/1  "<mag>"
  Bus Selector/1 -> Rate Transition/1  "<accel>"
  Bus Selector/2 -> Rate Transition1/1  "<gyro>"
  Demux2/3 -> Bus Assignment/11
  Demux2/2 -> Bus Assignment/10
  Demux/3 -> Bus Assignment/4
  Demux1/2 -> Bus Assignment/6
  Demux2/1 -> Bus Assignment/9
  Bus Assignment/1 -> Publish/1
  Demux1/4 -> Bus Assignment/8
  Demux1/1 -> Bus Assignment/5
  Demux/1 -> Bus Assignment/2
  Header Assignment/1 -> Bus Assignment/1
  Blank Message/1 -> Header Assignment/1

== system Simulation/ROS Output/Send Ping msg ==
  Mesure : Inport
  Blank Message : ros2lib/Blank Message  messageClass=Message  entityType=sonia_common_ros2/PingAngles  messageType=sonia_common_ros2/PingAngles  SampleTime=inf
  Bus Assignment : BusAssignment  AssignedSignals=heading,elevation
  Bus Selector : BusSelector  OutputSignals=Hydro Angles
  Demux : Demux  Outputs=3
  Publish : ros2lib/Publish  topicSource=Specify your own  topic=/proc_simulation/ping  messageType=sonia_common_ros2/PingAngles  QOSHistory=Keep last  QOSDepth=1  QOSReliability=Reliable  QOSDurability=Volatile  QOSDeadline=Inf  QOSLifespan=Inf  QOSLiveliness=Automatic  QOSLeaseDuration=Inf  QOSAvoidROSNamespaceConventions=off
  Terminator : Terminator
  Zero-Order Hold : ZeroOrderHold  SampleTime=simulation.sensors.depth.sampletime
  wires:
  Bus Assignment/1 -> Publish/1
  Demux/3 -> Terminator/1
  Zero-Order Hold/1 -> Demux/1
  Demux/2 -> Bus Assignment/3
  Demux/1 -> Bus Assignment/2
  Bus Selector/1 -> Zero-Order Hold/1  "<Hydro Angles>"
  Mesure/1 -> Bus Selector/1
  Blank Message/1 -> Bus Assignment/1

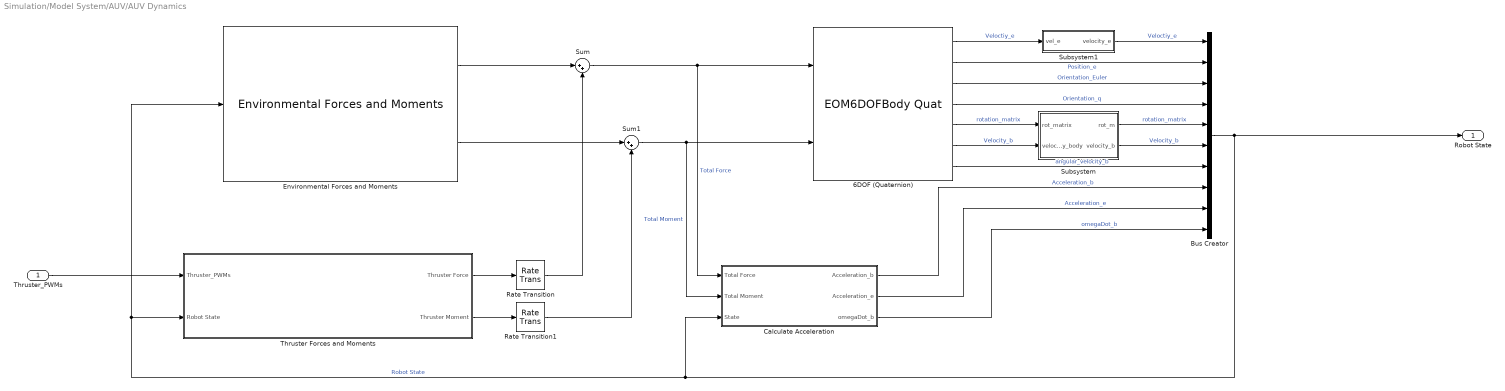
== system Simulation/Model System/AUV/AUV Dynamics ==
  Thruster_PWMs : Inport
  6DOF (Quaternion) : EOM6DOFBodyQuat  xme_0=AUV_pos  eul_0=AUV_orientation  mass_0=AUV_mass  inertia=AUV_inertia
  Bus Creator : BusCreator  Inputs=10
  Calculate Acceleration : Subsystem
  Environmental Forces and Moments : AUVLib/Environmental Forces and Moments  V=AUV_vol  h=AUV_height  mass=AUV_mass  CoB=AUV_cob  Hy=Simple  ang_coeff=ang_coeff  quad_coeff=quad_coeff  lin_coeff=lin_coeff  ang_coeff_c=ang_coeff_c  alphaR=alphaR  betaR=betaR  CX=CX  CY=CY  CZ=CZ  CMK=CMK  CMM=CMM  CMN=CMN  inputAxes=Body  cbar=1  b=1  S=1
  Rate Transition : RateTransition  OutPortSampleTime=0.05
  Rate Transition1 : RateTransition  OutPortSampleTime=0.05
  Subsystem : Subsystem
  Subsystem1 : Subsystem
  Sum : Sum  Inputs=|++
  Sum1 : Sum  Inputs=|++
  Thruster Forces and Moments : Subsystem
  Robot State : Outport
  wires:
  Rate Transition1/1 -> Sum1/2
  Rate Transition/1 -> Sum/2
  Environmental Forces and Moments/1 -> Sum/1
  Environmental Forces and Moments/2 -> Sum1/1
  Subsystem1/1(velocity_e) -> Bus Creator/1  "Veloctiy_e"
  Subsystem/1(rot_m) -> Bus Creator/5  "rotation_matrix"
  Subsystem/2(velocity_b) -> Bus Creator/6  "Velocity_b"
  6DOF (Quaternion)/6 -> Subsystem/2(velocity_body)  "Velocity_b"
  6DOF (Quaternion)/5 -> Subsystem/1(rot_matrix)  "rotation_matrix"
  6DOF (Quaternion)/2 -> Bus Creator/2  "Position_e"
  Bus Creator/1 -> Environmental Forces and Moments/1, Thruster Forces and Moments/2(Robot State), Calculate Acceleration/3(State), Robot State/1  "Robot State"
  6DOF (Quaternion)/4 -> Bus Creator/4  "Orientation_q"
  Calculate Acceleration/1(Acceleration_b) -> Bus Creator/8  "Acceleration_b"
  Thruster_PWMs/1 -> Thruster Forces and Moments/1(Thruster_PWMs)
  6DOF (Quaternion)/1 -> Subsystem1/1(vel_e)  "Veloctiy_e"
  Calculate Acceleration/2(Acceleration_e) -> Bus Creator/9  "Acceleration_e"
  Sum/1 -> Calculate Acceleration/1(Total Force), 6DOF (Quaternion)/1  "Total Force"
  6DOF (Quaternion)/7 -> Bus Creator/7  "angular_velocity_b"
  Calculate Acceleration/3(omegaDot_b) -> Bus Creator/10  "omegaDot_b"
  Thruster Forces and Moments/2(Thruster Moment) -> Rate Transition1/1
  Sum1/1 -> Calculate Acceleration/2(Total Moment), 6DOF (Quaternion)/2  "Total Moment"
  Thruster Forces and Moments/1(Thruster Force) -> Rate Transition/1
  6DOF (Quaternion)/3 -> Bus Creator/3  "Orientation_Euler"

== system Simulation/Model System/AUV/Actuators ==
  Robot State : Inport
  Launch_torpedo : Inport  Port=2
  drop_marker : Inport  Port=3
  Marker : Subsystem
  Tropedo : Subsystem
  Torpedo Pose : Outport
  marker_position : Outport  Port=2
  wires:
  Marker/1(marker_position) -> marker_position/1
  Tropedo/1(Torpedo Pose) -> Torpedo Pose/1
  Robot State/1 -> Tropedo/2(Robot State), Marker/1(robot_state)
  drop_marker/1 -> Marker/2(drop_marker)
  Launch_torpedo/1 -> Tropedo/1(launch_torpedo)

== system Simulation/Model System/AUV/Sensors ==
  Robot State : Inport
  Bus Creator : BusCreator  Inputs=11
  Bus Selector1 : BusSelector  OutputSignals=Velocity_b,Position_e,rotation_matrix
  Constant1 : Constant  Value=ref_mode  OutDataTypeStr=uint8
  Constant2 : Constant  Value=waterCurrent
  DVL : MATLAB Function  TreatAsAtomicUnit=on
  IMU Subsystem : Subsystem
  downward_camera : sim3dcameralib/Simulation 3D Camera  Priority=1  sensorTag=Sim3dSensor�  sensorId=1  sensorName=Sim3dSensor5  vehTagList={'Scene Origin'}  vehTag=Scene Origin  CoordinateSystem=ISO8855  mountLoc=Origin  offsetFlag=on  tmountOffset=d_cam_pos  extTmount=off  rmountOffset=d_orientation  extRmount=off  FocalLength=FocalLength  OpticalCenter=OpticalCenter  ImageSize=ImageSize  RadialDistortion=RadialDistortion  TangentialDistortion=TangentialDistortion  SensorSkew=0  VisualizeFieldOfView=off  FieldOfViewRange=61  DepthOutportEnabled=off  SemanticOutportEnabled=off  TransformOutportEnabled=off  SampleTime=0.1  mountPoint=[0 0 -0.26]  mountOrientation=[0 90 0]  aMode=3  ID=1
      settings: LibrarySourceBlock=drivingsim3d/Simulation 3D Camera
  forward_camera : sim3dcameralib/Simulation 3D Camera  Priority=1  sensorTag=Sim3dSensor�  sensorId=2  sensorName=Sim3dSensor6  vehTagList={'Scene Origin'}  vehTag=Scene Origin  CoordinateSystem=ISO8855  mountLoc=Origin  offsetFlag=on  tmountOffset=f_cam_pos  extTmount=off  rmountOffset=f_orientation  extRmount=off  FocalLength=FocalLength_f  OpticalCenter=OpticalCenter_f  ImageSize=ImageSize_f  RadialDistortion=RadialDistortion_f  TangentialDistortion=TangentialDistortion_f  SensorSkew=0  VisualizeFieldOfView=off  FieldOfViewRange=61  DepthOutportEnabled=on  SemanticOutportEnabled=off  TransformOutportEnabled=off  SampleTime=0.1  mountPoint=[0.5 0 0]  mountOrientation=[0 0 0]  aMode=6  ID=2
      settings: LibrarySourceBlock=robotsim3dlib/Simulation 3D Camera
  Sensor Values : Outport
  wires:
  forward_camera/2 -> Bus Creator/10  "forward_depth"
  IMU Subsystem/3(mag) -> Bus Creator/4
  IMU Subsystem/2(gyro) -> Bus Creator/3
  IMU Subsystem/1(accel) -> Bus Creator/2
  downward_camera/1 -> Bus Creator/11  "downward_camera"
  forward_camera/1 -> Bus Creator/9  "forward_camera"
  Bus Creator/1 -> Sensor Values/1
  DVL/4(reference) -> Bus Creator/8  "reference"
  DVL/3(vel_cov_diag_dvl) -> Bus Creator/7  "vel_cov_diag_dvl"
  DVL/2(altitude_dvl) -> Bus Creator/6  "altitude_dvl"
  DVL/1(vel_b_dvl) -> Bus Creator/5  "vel_b_dvl"
  Constant1/1 -> DVL/5(reference_mode)
  Constant2/1 -> DVL/4(v_current_e)
  Bus Selector1/3 -> DVL/3(rot_m)  "<rotation_matrix>"
  Bus Selector1/2 -> DVL/2(position_e), Bus Creator/1  "<Position_e>"
  Bus Selector1/1 -> DVL/1(body_vel)  "<Velocity_b>"
  Robot State/1 -> Bus Selector1/1, IMU Subsystem/1(Robot State)

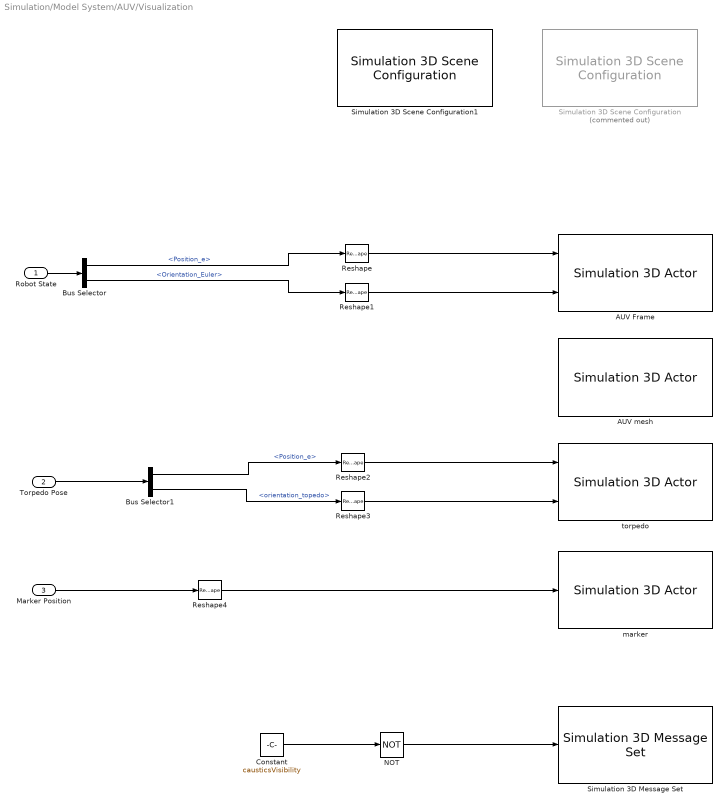
== system Simulation/Model System/AUV/Visualization ==
  Robot State : Inport
  Torpedo Pose : Inport  Port=2
  Marker Position : Inport  Port=3
  AUV Frame : sim3dlib/Simulation 3D Actor  Priority=1  ActorName=AUVframe  ParentName=Scene Origin  Operation=Create at setup  InitScriptText=|  SampleTime=-1  Translation=[0 0 0]  Rotation=[0 0 0]  Scale=[1 1 1]  InputsText=AUVframe.Translation AUVframe.Rotation  aMode=5  ActorTag=AUVframe  ActorType=Sim3dActor  ID=C
      | Actor.CoordinateSystem = 'AERO';
      | Actor.Collisions = false;
  AUV mesh : sim3dlib/Simulation 3D Actor  Priority=1  ActorName=Sim3dActor1  ParentName=AUVframe  Operation=Create at setup  InitScriptText=|  SampleTime=-1  Translation=[0 0 0]  Rotation=[0 0 0]  Scale=[1 1 1]  aMode=5  ActorTag=Sim3dActor1  ActorType=Sim3dActor  ID=1
      | Actor.CoordinateSystem = 'AERO';
      | % createShape(Actor, 'Cylinder', [1 0.5 0.5]);
      | Actor.Collisions = false;
  Bus Selector : BusSelector  OutputSignals=Position_e,Orientation_Euler
  Bus Selector1 : BusSelector  OutputSignals=Position_e,orientation_topedo
  Constant : Constant  Value=causticsVisibility  OutDataTypeStr=boolean
  NOT : Logic  Operator=NOT  IconShape=distinctive  AllPortsSameDT=off  OutDataTypeStr=boolean
  Reshape{,1..4} (5 alike) : Reshape  OutputDimensionality=Row vector (2-D)
  Simulation 3D Message Set : sim3dlib/Simulation 3D Message Set  Priority=-1  SigName=causticsVis  Ts=0.05  aMode=0
      settings: LibrarySourceBlock=aerolibsim3d/Simulation 3D Message Set
  Simulation 3D Scene Configuration : sim3dlib/Simulation 3D Scene Configuration  Priority=0  Commented=on  ProjectFormat=Unreal Executable  SceneDesc=Empty scene  ProjectName=/home/ubuntu/Téléchargements/RoboSub_pool_25b/Windows/AutoVrtlEnv.exe  ScenePath=/Game/Maps/RoboSub_pool  EnableOpenDRIVE=off  vehTagList={'AUVframe';'Custom';'Custom_pool';'Scene Origin';'Sim3dActor3';'marker';'torpedo'}  vehTag=Custom_pool  AttachedCameraRelativeTranslation=[0 0 0]  FreeCameraDefaultInitialTranslation=[-6, 0, 2]  AttachedCameraRelativeRotation=[0 0 0]  FreeCameraDefaultInitialRotation=[0, -15, 0]  ViewpointName=Custom_pool  FreeCameraInitialTranslation=[-150 -142 2.5]  ViewpointTranslation=[0 0 0]  FreeCameraInitialRotation=[0 0 0]  ViewpointRotation=[0 0 0]  OpVisEn=off  Ts=.01  EnableWindow=on  EnableRemoteAccess=off  EnableWeather=off  SunAzimuth=90  SunAltitude=40.0  EnableGeospatialSun=off  Latitude=0  Longitude=0  Date=2023-01-01  Time=10:30:00  GeoTimeZone=-5.0  SunDaylightSaving=off  wind=1  clouds=10  EnableVolumetricClouds=off  CloudCoverage=0  CloudAltitude=6  fog=0  rain=0  RaindropsEffect=off  SnowDensity=0  EnableGeospatial=off  TilesetSource=Earth terrain  UseTrueOrigin=off  OriginHeight=200  OriginLatitude=40.744652  OriginLongitude=-73.988864  MapStyle=Aerial  AdditionalAssetIDs=[]  UseAdvancedSunSky=off  SolarTime=11  TimeZone=-5  Day=21  Month=9  Year=2022  UseDaylightSavingTime=on  DSTStartDay=10  DSTStartMonth=3  DSTEndDay=3  DSTEndMonth=11  DSTSwitchHour=2  sensorTag=MainCamera1  sensorId=1  sensorName=MainCamera1  mountLoc=Origin  offsetFlag=off  tmountOffset=[0, 0, 0]  rmountOffset=[0, 0, 0]  HorizontalResolution=1280  VerticalResolution=720  HorizontalFOV=60  mountPoint=[0 0 0]  mountOrientation=[0 0 0]  aMode=5  ID=1  GeoTrigger=Inactive  ViewNameList={'Custom', 'Custom_pool'}  ViewTranslationList={'[-100 -100 1]', '[-150 -142 2.5]'}  ViewRotationList={'[0 0 0]', '[0 0 0]'}
      settings: LibrarySourceBlock=sl3dlib/Simulation 3D/Environment/Simulation 3D Scene Configuration
  Simulation 3D Scene Configuration1 : sim3dlib/Simulation 3D Scene Configuration  Priority=0  ProjectFormat=Default Scenes  SceneDesc=Straight road  ProjectName=/usr/local/MATLAB/R2025b/toolbox/shared/sim3d_projects/automotive_project_linux/UE/LinuxNoEditor/VehicleSimulation.sh  ScenePath=/Game/Maps/RoboSub_pool  EnableOpenDRIVE=off  vehTagList={'AUVframe';'Custom';'Custom_pool';'Scene Origin';'Sim3dActor1'}  vehTag=Custom_pool  AttachedCameraRelativeTranslation=[0 0 0]  FreeCameraDefaultInitialTranslation=[-6, 0, 2]  AttachedCameraRelativeRotation=[0 0 0]  FreeCameraDefaultInitialRotation=[0, -15, 0]  ViewpointName=Custom_pool  FreeCameraInitialTranslation=[-150 -142 2.5]  ViewpointTranslation=[0 0 0]  FreeCameraInitialRotation=[0 0 0]  ViewpointRotation=[0 0 0]  OpVisEn=off  Ts=.1  EnableWindow=on  EnableRemoteAccess=off  EnableWeather=off  SunAzimuth=90  SunAltitude=40.0  EnableGeospatialSun=off  Latitude=0  Longitude=0  Date=2023-01-01  Time=10:30:00  GeoTimeZone=-5.0  SunDaylightSaving=off  wind=1  clouds=10  EnableVolumetricClouds=off  CloudCoverage=0  CloudAltitude=6  fog=0  rain=0  RaindropsEffect=off  SnowDensity=0  EnableGeospatial=off  TilesetSource=Earth terrain  UseTrueOrigin=off  OriginHeight=200  OriginLatitude=40.744652  OriginLongitude=-73.988864  MapStyle=Aerial  AdditionalAssetIDs=[]  UseAdvancedSunSky=off  SolarTime=11  TimeZone=-5  Day=21  Month=9  Year=2022  UseDaylightSavingTime=on  DSTStartDay=10  DSTStartMonth=3  DSTEndDay=3  DSTEndMonth=11  DSTSwitchHour=2  sensorTag=MainCamera2  sensorId=1  sensorName=MainCamera2  mountLoc=Origin  offsetFlag=off  tmountOffset=[0, 0, 0]  rmountOffset=[0, 0, 0]  HorizontalResolution=1280  VerticalResolution=720  HorizontalFOV=60  mountPoint=[0 0 0]  mountOrientation=[0 0 0]  aMode=5  ID=1  GeoTrigger=Inactive  ViewNameList={'Custom', 'Custom_pool'}  ViewTranslationList={'[-100 -100 1]', '[-150 -142 2.5]'}  ViewRotationList={'[0 0 0]', '[0 0 0]'}
      settings: LibrarySourceBlock=sl3dlib/Simulation 3D/Environment/Simulation 3D Scene Configuration
  marker : sim3dlib/Simulation 3D Actor  Priority=1  ActorName=marker  ParentName=Scene Origin  Operation=Create at setup  InitScriptText=|  SampleTime=-1  Translation=[0 0 0]  Rotation=[0 0 pi/2]  Scale=[1 1 1]  InputsText=marker.Translation  aMode=5  ActorTag=marker  ActorType=Sim3dActor  ID=C
      | % Reserved keywords:
      | % - Actor : handle to this actor object
      | % - World : handle to the world object
      | 
      | % Examples:
      | 
      | % Create a primitive geometry (optional)
      | % createShape(Actor, 'box', [1 1 1]);
      | 
      | % Initialize values (optional)
      | % Actor.Physics = true;
      | % Actor.Color = [1 0 0];
      | Actor.CoordinateSystem = 'AERO';
      | createShape(Actor, 'sphere', [0.1 0.1 0.1]);
      | Actor.Color = [0 1 0];
  torpedo : sim3dlib/Simulation 3D Actor  Priority=1  ActorName=torpedo  ParentName=SceneOrigin  Operation=Create at setup  InitScriptText=|  SampleTime=-1  Translation=[0 0.27 0]  Rotation=[0 0 pi/2]  Scale=[1 1 1]  InputsText=torpedo.Translation torpedo.Rotation  aMode=5  ActorTag=torpedo  ActorType=Sim3dActor  ID=C
      | % Reserved keywords:
      | % - Actor : handle to this actor object
      | % - World : handle to the world object
      | 
      | % Examples:
      | 
      | % Create a primitive geometry (optional)
      | % createShape(Actor, 'box', [1 1 1]);
      | 
      | % Initialize values (optional)
      | % Actor.Physics = true;
      | % Actor.Color = [1 0 0];
      | Actor.CoordinateSystem = 'AERO';
      | createShape(Actor, 'box', [0.15 0.01 0.01]);
      | Actor.Color = [1 0 0];
  wires:
  NOT/1 -> Simulation 3D Message Set/1
  Constant/1 -> NOT/1
  Bus Selector1/2 -> Reshape3/1  "<orientation_topedo>"
  Reshape1/1 -> AUV Frame/2
  Reshape4/1 -> marker/1
  Marker Position/1 -> Reshape4/1
  Bus Selector1/1 -> Reshape2/1  "<Position_e>"
  Reshape3/1 -> torpedo/2
  Reshape2/1 -> torpedo/1
  Reshape/1 -> AUV Frame/1
  Bus Selector/2 -> Reshape1/1  "<Orientation_Euler>"
  Bus Selector/1 -> Reshape/1  "<Position_e>"
  Robot State/1 -> Bus Selector/1
  Torpedo Pose/1 -> Bus Selector1/1

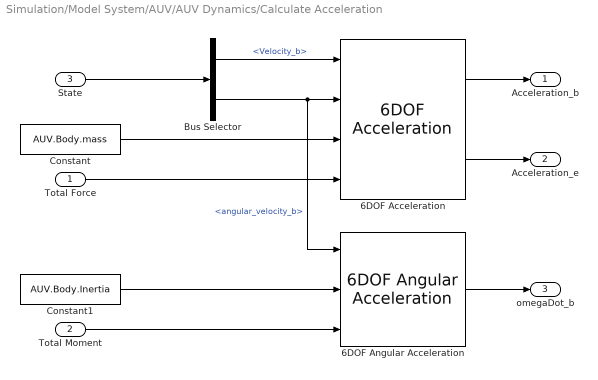
== system Simulation/Model System/AUV/AUV Dynamics/Calculate Acceleration ==
  Total Force : Inport
  Total Moment : Inport  Port=2
  State : Inport  Port=3
  6DOF Acceleration : aerolib6dof2/6DOF Acceleration  units=Metric (MKS)  mtype=Fixed  vre_flag=off
  6DOF Angular Acceleration : aerolib6dof2/6DOF Angular Acceleration  units=Metric (MKS)  mtype=Fixed
  Bus Selector : BusSelector  OutputSignals=Velocity_b,angular_velocity_b
  Constant : Constant  Value=AUV.Body.mass
  Constant1 : Constant  Value=AUV.Body.Inertia
  Acceleration_b : Outport
  Acceleration_e : Outport  Port=2
  omegaDot_b : Outport  Port=3
  wires:
  6DOF Acceleration/2 -> Acceleration_e/1
  6DOF Angular Acceleration/1 -> omegaDot_b/1
  6DOF Acceleration/1 -> Acceleration_b/1
  Constant1/1 -> 6DOF Angular Acceleration/2
  Bus Selector/1 -> 6DOF Acceleration/1  "<Velocity_b>"
  Total Force/1 -> 6DOF Acceleration/4
  State/1 -> Bus Selector/1
  Total Moment/1 -> 6DOF Angular Acceleration/3
  Bus Selector/2 -> 6DOF Acceleration/2, 6DOF Angular Acceleration/1  "<angular_velocity_b>"
  Constant/1 -> 6DOF Acceleration/3

== system Simulation/Model System/AUV/AUV Dynamics/Subsystem ==
  rot_matrix : Inport
  velocity_body : Inport  Port=2
  Matrix Multiply : Product  Multiplication=Matrix(*)
  Sum : Sum  Inputs=|-+
  currentVelocity_e : Constant  Value=waterCurrent
  rot_m : Outport
  velocity_b : Outport  Port=2
  wires:
  Matrix Multiply/1 -> Sum/1
  Sum/1 -> velocity_b/1
  velocity_body/1 -> Sum/2
  rot_matrix/1 -> rot_m/1, Matrix Multiply/1
  currentVelocity_e/1 -> Matrix Multiply/2

== system Simulation/Model System/AUV/AUV Dynamics/Subsystem1 ==
  vel_e : Inport
  Sum : Sum  Inputs=|++
  currentVelocity : Constant  Value=waterCurrent
  velocity_e : Outport
  wires:
  currentVelocity/1 -> Sum/2
  Sum/1 -> velocity_e/1
  vel_e/1 -> Sum/1

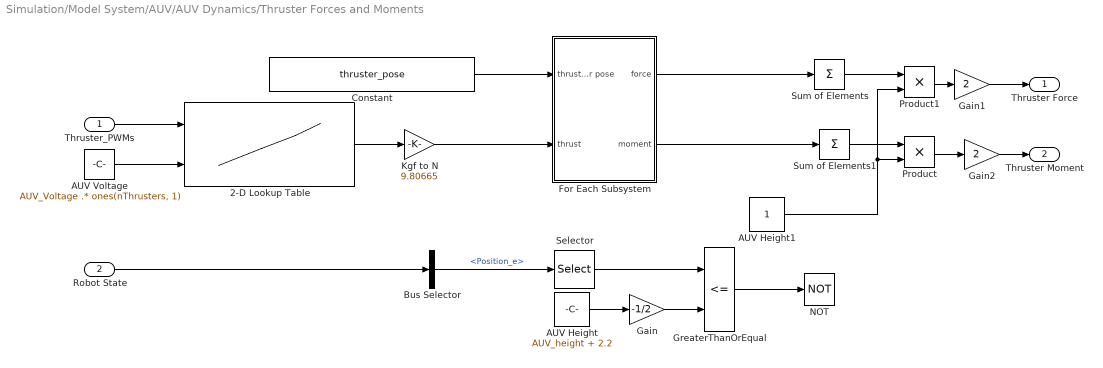
== system Simulation/Model System/AUV/AUV Dynamics/Thruster Forces and Moments ==
  Thruster_PWMs : Inport
  Robot State : Inport  Port=2
  2-D Lookup Table : Lookup_n-D  BreakpointsForDimension1=T200.pwm  BreakpointsForDimension2=T200.voltages  Table=T200.thrust  InternalRulePriority=Speed  RndMeth=Simplest
      settings: InputPortMap=u0,u1
  AUV Height : Constant  Value=AUV_height + 2.2
  AUV Height1 : Constant
  AUV Voltage : Constant  Value=AUV_Voltage .* ones(nThrusters, 1)
  Bus Selector : BusSelector  OutputSignals=Position_e
  Constant : Constant  Value=thruster_pose
  For Each Subsystem : Subsystem  TreatAsAtomicUnit=on
  Gain : Gain  Gain=-1/2
  Gain1 : Gain  Gain=2
  Gain2 : Gain  Gain=2
  GreaterThanOrEqual : RelationalOperator  Operator=<=  OutDataTypeStr=boolean  RndMeth=Simplest  InputSameDT=off
  Kgf to N : Gain  Gain=9.80665
  NOT : Logic  Operator=NOT  IconShape=distinctive  AllPortsSameDT=off  OutDataTypeStr=boolean
  Product : Product
  Product1 : Product
  Selector : Selector  InputPortWidth=3  IndexOptions=Index vector (dialog)  Indices=[3]  OutputSizes=1
  Sum of Elements : Sum  Inputs=+  CollapseMode=Specified dimension
  Sum of Elements1 : Sum  Inputs=+  CollapseMode=Specified dimension
  Thruster Force : Outport
  Thruster Moment : Outport  Port=2
  wires:
  Gain2/1 -> Thruster Moment/1
  Gain1/1 -> Thruster Force/1
  AUV Height1/1 -> Product/2, Product1/2
  Kgf to N/1 -> For Each Subsystem/2(thrust)
  AUV Voltage/1 -> 2-D Lookup Table/2
  2-D Lookup Table/1 -> Kgf to N/1
  Thruster_PWMs/1 -> 2-D Lookup Table/1
  GreaterThanOrEqual/1 -> NOT/1
  Product/1 -> Gain2/1
  Sum of Elements1/1 -> Product/1
  Product1/1 -> Gain1/1
  Sum of Elements/1 -> Product1/1
  Gain/1 -> GreaterThanOrEqual/2
  Selector/1 -> GreaterThanOrEqual/1
  AUV Height/1 -> Gain/1
  Bus Selector/1 -> Selector/1  "<Position_e>"
  Robot State/1 -> Bus Selector/1
  For Each Subsystem/1(force) -> Sum of Elements/1
  For Each Subsystem/2(moment) -> Sum of Elements1/1
  Constant/1 -> For Each Subsystem/1(thruster pose)

== system Simulation/Model System/AUV/Actuators/Marker ==
  robot_state : Inport
  drop_marker : Inport  Port=2
  Get Inital state : AUVLib/Get Inital state  SystemSampleTime=-1  VariantActivationTime=update diagram  EmptyChoice=off  PassThrough=off  PassThroughVariantControl=(default)  EmptyChoiceVariantControl=(default)  AllowFlexibleInterface=on  Latency=0  AutoFrameSizeCalculation=off
  Marker Dynamics : Subsystem  TreatAsAtomicUnit=on
  marker_position : Outport
  wires:
  Marker Dynamics/1(marker_position) -> marker_position/1
  drop_marker/1 -> Marker Dynamics/Enable, Get Inital state/Trigger
  Get Inital state/1 -> Marker Dynamics/1(Initial_state)
  robot_state/1 -> Get Inital state/1

== system Simulation/Model System/AUV/Actuators/Tropedo ==
  launch_torpedo : Inport
  Robot State : Inport  Port=2
  Get Inital state : AUVLib/Get Inital state  SystemSampleTime=-1  VariantActivationTime=update diagram  EmptyChoice=off  PassThrough=off  PassThroughVariantControl=(default)  EmptyChoiceVariantControl=(default)  AllowFlexibleInterface=on  Latency=0  AutoFrameSizeCalculation=off
  Torpedo Dynamics : Subsystem  TreatAsAtomicUnit=on
  Torpedo Pose : Outport
  wires:
  Torpedo Dynamics/1(Torpedo Pose) -> Torpedo Pose/1
  Robot State/1 -> Get Inital state/1
  launch_torpedo/1 -> Torpedo Dynamics/Enable, Get Inital state/Trigger
  Get Inital state/1 -> Torpedo Dynamics/1(Initial_state)
